simulink model "Q1"  (R2016b)
settings: Solver=VariableStepAuto  StartTime=0.0  StopTime=totaltime  RelTol=1e-3
undefined symbols (not defined in the file): b, st
libraries: xbsIndex_r4 x131
settings Model: Creator=rm101  LastModifiedBy=rm101

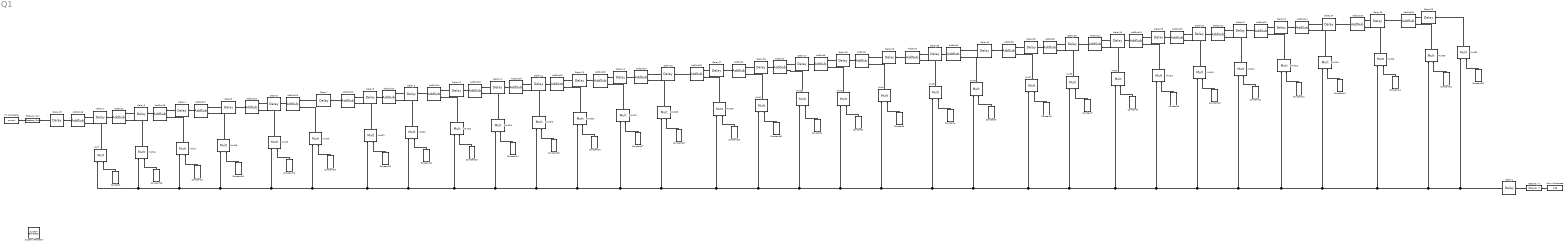
== system Q1 ==
  " System Generator" : xbsIndex_r4/ System Generator  Tag=genX  xilinxfamily=zynq  part=xc7z020  speed=-1  package=clg484  synthesis_tool=Vivado  clock_wrapper=Clock Enables  directory=E:/yg/lab1/generator/Q1_new2  proj_type=Vivado  Synth_file=Vivado Synthesis Defaults  Impl_file=Vivado Implementation Defaults  testbench=off  simulink_period=st  sysclk_period=st*10e6  dcm_input_clock_period=10  incr_netlist=off  trim_vbits=Everywhere in SubSystem  dbl_ovrd=According to Block Masks  core_generation=According to Block Masks  run_coregen=off  deprecated_control=off  eval_field=0  block_type=sysgen
  AddSub{1..31} (31 alike) : xbsIndex_r4/AddSub  mode=Addition  use_carryin=off  use_carryout=off  en=off  latency=0  precision=Full  arith_type=Unsigned  n_bits=16  bin_pt=14  quantization=Truncate  overflow=Wrap  use_behavioral_HDL=off  hw_selection=Fabric  pipelined=off  dbl_ovrd=off  block_type=addsub
  Constant : xbsIndex_r4/Constant  const=b(1)  gui_display_data_type=Fixed-point  arith_type=Signed (2's comp)  n_bits=W  bin_pt=D  preci_type=Single  exp_width=8  frac_width=24  explicit_period=off  period=1  equ=P=C  opselect=C  inp2=PCIN>>17  opr=+  inp1=P  carry=CIN  dbl_ovrd=off  block_type=constant
  Constant1 : xbsIndex_r4/Constant  const=b(17)  gui_display_data_type=Fixed-point  arith_type=Signed (2's comp)  n_bits=W  bin_pt=D  preci_type=Single  exp_width=8  frac_width=24  explicit_period=off  period=1  equ=P=C  opselect=C  inp2=PCIN>>17  opr=+  inp1=P  carry=CIN  dbl_ovrd=off  block_type=constant
  Constant10 : xbsIndex_r4/Constant  const=b(26)  gui_display_data_type=Fixed-point  arith_type=Signed (2's comp)  n_bits=W  bin_pt=D  preci_type=Single  exp_width=8  frac_width=24  explicit_period=off  period=1  equ=P=C  opselect=C  inp2=PCIN>>17  opr=+  inp1=P  carry=CIN  dbl_ovrd=off  block_type=constant
  Constant11 : xbsIndex_r4/Constant  const=b(27)  gui_display_data_type=Fixed-point  arith_type=Signed (2's comp)  n_bits=W  bin_pt=D  preci_type=Single  exp_width=8  frac_width=24  explicit_period=off  period=1  equ=P=C  opselect=C  inp2=PCIN>>17  opr=+  inp1=P  carry=CIN  dbl_ovrd=off  block_type=constant
  Constant12 : xbsIndex_r4/Constant  const=b(28)  gui_display_data_type=Fixed-point  arith_type=Signed (2's comp)  n_bits=W  bin_pt=D  preci_type=Single  exp_width=8  frac_width=24  explicit_period=off  period=1  equ=P=C  opselect=C  inp2=PCIN>>17  opr=+  inp1=P  carry=CIN  dbl_ovrd=off  block_type=constant
  Constant13 : xbsIndex_r4/Constant  const=b(29)  gui_display_data_type=Fixed-point  arith_type=Signed (2's comp)  n_bits=W  bin_pt=D  preci_type=Single  exp_width=8  frac_width=24  explicit_period=off  period=1  equ=P=C  opselect=C  inp2=PCIN>>17  opr=+  inp1=P  carry=CIN  dbl_ovrd=off  block_type=constant
  Constant14 : xbsIndex_r4/Constant  const=b(30)  gui_display_data_type=Fixed-point  arith_type=Signed (2's comp)  n_bits=W  bin_pt=D  preci_type=Single  exp_width=8  frac_width=24  explicit_period=off  period=1  equ=P=C  opselect=C  inp2=PCIN>>17  opr=+  inp1=P  carry=CIN  dbl_ovrd=off  block_type=constant
  Constant16 : xbsIndex_r4/Constant  const=b(2)  gui_display_data_type=Fixed-point  arith_type=Signed (2's comp)  n_bits=W  bin_pt=D  preci_type=Single  exp_width=8  frac_width=24  explicit_period=off  period=1  equ=P=C  opselect=C  inp2=PCIN>>17  opr=+  inp1=P  carry=CIN  dbl_ovrd=off  block_type=constant
  Constant17 : xbsIndex_r4/Constant  const=b(3)  gui_display_data_type=Fixed-point  arith_type=Signed (2's comp)  n_bits=W  bin_pt=D  preci_type=Single  exp_width=8  frac_width=24  explicit_period=off  period=1  equ=P=C  opselect=C  inp2=PCIN>>17  opr=+  inp1=P  carry=CIN  dbl_ovrd=off  block_type=constant
  Constant18 : xbsIndex_r4/Constant  const=b(4)  gui_display_data_type=Fixed-point  arith_type=Signed (2's comp)  n_bits=W  bin_pt=D  preci_type=Single  exp_width=8  frac_width=24  explicit_period=off  period=1  equ=P=C  opselect=C  inp2=PCIN>>17  opr=+  inp1=P  carry=CIN  dbl_ovrd=off  block_type=constant
  Constant19 : xbsIndex_r4/Constant  const=b(5)  gui_display_data_type=Fixed-point  arith_type=Signed (2's comp)  n_bits=W  bin_pt=D  preci_type=Single  exp_width=8  frac_width=24  explicit_period=off  period=1  equ=P=C  opselect=C  inp2=PCIN>>17  opr=+  inp1=P  carry=CIN  dbl_ovrd=off  block_type=constant
  Constant2 : xbsIndex_r4/Constant  const=b(18)  gui_display_data_type=Fixed-point  arith_type=Signed (2's comp)  n_bits=W  bin_pt=D  preci_type=Single  exp_width=8  frac_width=24  explicit_period=off  period=1  equ=P=C  opselect=C  inp2=PCIN>>17  opr=+  inp1=P  carry=CIN  dbl_ovrd=off  block_type=constant
  Constant20 : xbsIndex_r4/Constant  const=b(6)  gui_display_data_type=Fixed-point  arith_type=Signed (2's comp)  n_bits=W  bin_pt=D  preci_type=Single  exp_width=8  frac_width=24  explicit_period=off  period=1  equ=P=C  opselect=C  inp2=PCIN>>17  opr=+  inp1=P  carry=CIN  dbl_ovrd=off  block_type=constant
  Constant21 : xbsIndex_r4/Constant  const=b(7)  gui_display_data_type=Fixed-point  arith_type=Signed (2's comp)  n_bits=W  bin_pt=D  preci_type=Single  exp_width=8  frac_width=24  explicit_period=off  period=1  equ=P=C  opselect=C  inp2=PCIN>>17  opr=+  inp1=P  carry=CIN  dbl_ovrd=off  block_type=constant
  Constant22 : xbsIndex_r4/Constant  const=b(8)  gui_display_data_type=Fixed-point  arith_type=Signed (2's comp)  n_bits=W  bin_pt=D  preci_type=Single  exp_width=8  frac_width=24  explicit_period=off  period=1  equ=P=C  opselect=C  inp2=PCIN>>17  opr=+  inp1=P  carry=CIN  dbl_ovrd=off  block_type=constant
  Constant23 : xbsIndex_r4/Constant  const=b(9)  gui_display_data_type=Fixed-point  arith_type=Signed (2's comp)  n_bits=W  bin_pt=D  preci_type=Single  exp_width=8  frac_width=24  explicit_period=off  period=1  equ=P=C  opselect=C  inp2=PCIN>>17  opr=+  inp1=P  carry=CIN  dbl_ovrd=off  block_type=constant
  Constant24 : xbsIndex_r4/Constant  const=b(10)  gui_display_data_type=Fixed-point  arith_type=Signed (2's comp)  n_bits=W  bin_pt=D  preci_type=Single  exp_width=8  frac_width=24  explicit_period=off  period=1  equ=P=C  opselect=C  inp2=PCIN>>17  opr=+  inp1=P  carry=CIN  dbl_ovrd=off  block_type=constant
  Constant25 : xbsIndex_r4/Constant  const=b(11)  gui_display_data_type=Fixed-point  arith_type=Signed (2's comp)  n_bits=W  bin_pt=D  preci_type=Single  exp_width=8  frac_width=24  explicit_period=off  period=1  equ=P=C  opselect=C  inp2=PCIN>>17  opr=+  inp1=P  carry=CIN  dbl_ovrd=off  block_type=constant
  Constant26 : xbsIndex_r4/Constant  const=b(12)  gui_display_data_type=Fixed-point  arith_type=Signed (2's comp)  n_bits=W  bin_pt=D  preci_type=Single  exp_width=8  frac_width=24  explicit_period=off  period=1  equ=P=C  opselect=C  inp2=PCIN>>17  opr=+  inp1=P  carry=CIN  dbl_ovrd=off  block_type=constant
  Constant27 : xbsIndex_r4/Constant  const=b(13)  gui_display_data_type=Fixed-point  arith_type=Signed (2's comp)  n_bits=W  bin_pt=D  preci_type=Single  exp_width=8  frac_width=24  explicit_period=off  period=1  equ=P=C  opselect=C  inp2=PCIN>>17  opr=+  inp1=P  carry=CIN  dbl_ovrd=off  block_type=constant
  Constant28 : xbsIndex_r4/Constant  const=b(14)  gui_display_data_type=Fixed-point  arith_type=Signed (2's comp)  n_bits=W  bin_pt=D  preci_type=Single  exp_width=8  frac_width=24  explicit_period=off  period=1  equ=P=C  opselect=C  inp2=PCIN>>17  opr=+  inp1=P  carry=CIN  dbl_ovrd=off  block_type=constant
  Constant29 : xbsIndex_r4/Constant  const=b(15)  gui_display_data_type=Fixed-point  arith_type=Signed (2's comp)  n_bits=W  bin_pt=D  preci_type=Single  exp_width=8  frac_width=24  explicit_period=off  period=1  equ=P=C  opselect=C  inp2=PCIN>>17  opr=+  inp1=P  carry=CIN  dbl_ovrd=off  block_type=constant
  Constant3 : xbsIndex_r4/Constant  const=b(19)  gui_display_data_type=Fixed-point  arith_type=Signed (2's comp)  n_bits=W  bin_pt=D  preci_type=Single  exp_width=8  frac_width=24  explicit_period=off  period=1  equ=P=C  opselect=C  inp2=PCIN>>17  opr=+  inp1=P  carry=CIN  dbl_ovrd=off  block_type=constant
  Constant30 : xbsIndex_r4/Constant  const=b(16)  gui_display_data_type=Fixed-point  arith_type=Signed (2's comp)  n_bits=W  bin_pt=D  preci_type=Single  exp_width=8  frac_width=24  explicit_period=off  period=1  equ=P=C  opselect=C  inp2=PCIN>>17  opr=+  inp1=P  carry=CIN  dbl_ovrd=off  block_type=constant
  Constant31 : xbsIndex_r4/Constant  const=b(31)  gui_display_data_type=Fixed-point  arith_type=Signed (2's comp)  n_bits=W  bin_pt=D  preci_type=Single  exp_width=8  frac_width=24  explicit_period=off  period=1  equ=P=C  opselect=C  inp2=PCIN>>17  opr=+  inp1=P  carry=CIN  dbl_ovrd=off  block_type=constant
  Constant32 : xbsIndex_r4/Constant  const=b(32)  gui_display_data_type=Fixed-point  arith_type=Signed (2's comp)  n_bits=W  bin_pt=D  preci_type=Single  exp_width=8  frac_width=24  explicit_period=off  period=1  equ=P=C  opselect=C  inp2=PCIN>>17  opr=+  inp1=P  carry=CIN  dbl_ovrd=off  block_type=constant
  Constant4 : xbsIndex_r4/Constant  const=b(20)  gui_display_data_type=Fixed-point  arith_type=Signed (2's comp)  n_bits=W  bin_pt=D  preci_type=Single  exp_width=8  frac_width=24  explicit_period=off  period=1  equ=P=C  opselect=C  inp2=PCIN>>17  opr=+  inp1=P  carry=CIN  dbl_ovrd=off  block_type=constant
  Constant5 : xbsIndex_r4/Constant  const=b(21)  gui_display_data_type=Fixed-point  arith_type=Signed (2's comp)  n_bits=W  bin_pt=D  preci_type=Single  exp_width=8  frac_width=24  explicit_period=off  period=1  equ=P=C  opselect=C  inp2=PCIN>>17  opr=+  inp1=P  carry=CIN  dbl_ovrd=off  block_type=constant
  Constant6 : xbsIndex_r4/Constant  const=b(22)  gui_display_data_type=Fixed-point  arith_type=Signed (2's comp)  n_bits=W  bin_pt=D  preci_type=Single  exp_width=8  frac_width=24  explicit_period=off  period=1  equ=P=C  opselect=C  inp2=PCIN>>17  opr=+  inp1=P  carry=CIN  dbl_ovrd=off  block_type=constant
  Constant7 : xbsIndex_r4/Constant  const=b(23)  gui_display_data_type=Fixed-point  arith_type=Signed (2's comp)  n_bits=W  bin_pt=D  preci_type=Single  exp_width=8  frac_width=24  explicit_period=off  period=1  equ=P=C  opselect=C  inp2=PCIN>>17  opr=+  inp1=P  carry=CIN  dbl_ovrd=off  block_type=constant
  Constant8 : xbsIndex_r4/Constant  const=b(24)  gui_display_data_type=Fixed-point  arith_type=Signed (2's comp)  n_bits=W  bin_pt=D  preci_type=Single  exp_width=8  frac_width=24  explicit_period=off  period=1  equ=P=C  opselect=C  inp2=PCIN>>17  opr=+  inp1=P  carry=CIN  dbl_ovrd=off  block_type=constant
  Constant9 : xbsIndex_r4/Constant  const=b(25)  gui_display_data_type=Fixed-point  arith_type=Signed (2's comp)  n_bits=W  bin_pt=D  preci_type=Single  exp_width=8  frac_width=24  explicit_period=off  period=1  equ=P=C  opselect=C  inp2=PCIN>>17  opr=+  inp1=P  carry=CIN  dbl_ovrd=off  block_type=constant
  Delay{1..33} (33 alike) : xbsIndex_r4/Delay  rst=off  infoeditControl=Selection of Reset will increase slice count due to use of real FFs and instead of SRLs  en=off  latency=1  reg_retiming=off  dbl_ovrd=off  block_type=delay
  From Workspace : FromWorkspace  VariableName=sig3  SampleTime=0  Interpolate=off  OutputAfterFinalValue=Holding final value
  Gateway In : xbsIndex_r4/Gateway In  gui_display_data_type=Fixed-point  arith_type="Signed  (2's comp)"  n_bits=W  bin_pt=D  preci_type=Single  exp_width=8  frac_width=24  rows=1  columns=1  quantization="Round  (unbiased: +/- Inf)"  overflow=Flag as error  period=st  UseAsADC=off  ADCChannel='1'  interface=None  automatic_assignment=on  address_offset=hex2dec('00')  intf_name=''  intf_description=''  default_value=0  timing_constraint=None  locs_specified=off  LOCs={}  io_standard={}  inherit_from_input=off  hdl_port=on  dbl_ovrd=off  block_type=gatewayin
  Gateway Out : xbsIndex_r4/Gateway Out  inherit_from_input=off  hdl_port=on  rows=1  columns=1  UseAsDAC=off  DACChannel='1'  interface=None  automatic_assignment=on  address_offset=hex2dec('00')  intf_name=''  intf_description=''  timing_constraint=None  locs_specified=off  LOCs={}  io_standard={}  block_type=gatewayout
  Mult{,1..30,32} (32 alike) : xbsIndex_r4/Mult  precision=User Defined  arith_type="Signed  (2's comp)"  n_bits=W  bin_pt=D  quantization="Round  (unbiased: +/- Inf)"  overflow=Flag as error  en=off  latency=0  use_behavioral_HDL=off  opt=Speed  use_embedded=on  optimum_pipeline=off  pipeline=on  dbl_ovrd=off  use_rpm=on  placement_style=Triangular  block_type=mult
  To Workspace : ToWorkspace  VariableName=simout  SaveFormat=Timeseries  SampleTime=-1
  wires:
  Constant/1 -> Mult/2
  Gateway Out/1 -> To Workspace/1
  From Workspace/1 -> Gateway In/1
  Delay15/1 -> Gateway Out/1
  AddSub16/1 -> Delay15/1
  Mult/1 -> AddSub16/2
  Constant16/1 -> Mult16/2
  Mult16/1 -> AddSub1/2
  AddSub1/1 -> Delay2/1
  Constant17/1 -> Mult17/2
  Mult17/1 -> AddSub18/2
  Constant18/1 -> Mult18/2
  Mult18/1 -> AddSub17/2
  AddSub17/1 -> Delay4/1
  AddSub18/1 -> Delay3/1
  Constant19/1 -> Mult19/2
  Mult19/1 -> AddSub20/2
  Constant20/1 -> Mult20/2
  Mult20/1 -> AddSub19/2
  AddSub19/1 -> Delay6/1
  AddSub20/1 -> Delay5/1
  Constant21/1 -> Mult21/2
  Mult21/1 -> AddSub22/2
  Constant22/1 -> Mult22/2
  Mult22/1 -> AddSub21/2
  AddSub21/1 -> Delay8/1
  AddSub22/1 -> Delay7/1
  Constant23/1 -> Mult23/2
  Mult23/1 -> AddSub24/2
  Constant24/1 -> Mult24/2
  Mult24/1 -> AddSub23/2
  AddSub23/1 -> Delay10/1
  Constant25/1 -> Mult25/2
  Mult25/1 -> AddSub26/2
  Constant26/1 -> Mult26/2
  Mult26/1 -> AddSub25/2
  AddSub25/1 -> Delay12/1
  AddSub26/1 -> Delay11/1
  Constant27/1 -> Mult27/2
  Mult27/1 -> AddSub28/2
  Constant28/1 -> Mult28/2
  Mult28/1 -> AddSub27/2
  AddSub27/1 -> Delay14/1
  AddSub28/1 -> Delay13/1
  Constant29/1 -> Mult29/2
  Mult29/1 -> AddSub30/2
  AddSub30/1 -> Delay16/1
  AddSub24/1 -> Delay9/1
  Gateway In/1 -> Delay1/1
  Delay2/1 -> AddSub16/1
  Delay3/1 -> AddSub1/1
  Delay4/1 -> AddSub18/1
  Delay5/1 -> AddSub17/1
  Delay6/1 -> AddSub20/1
  Delay7/1 -> AddSub19/1
  Delay8/1 -> AddSub22/1
  Delay9/1 -> AddSub21/1
  Delay10/1 -> AddSub24/1
  Delay11/1 -> AddSub23/1
  Delay12/1 -> AddSub26/1
  Delay13/1 -> AddSub25/1
  Delay14/1 -> AddSub28/1
  Delay16/1 -> AddSub27/1
  Delay17/1 -> AddSub30/1
  Constant30/1 -> Mult1/2
  ? -> ?
  AddSub3/1 -> Delay17/1
  Mult1/1 -> AddSub3/2
  Constant1/1 -> Mult2/2
  Mult2/1 -> AddSub2/2
  AddSub2/1 -> Delay26/1
  Constant2/1 -> Mult3/2
  Mult3/1 -> AddSub5/2
  Constant3/1 -> Mult4/2
  Mult4/1 -> AddSub4/2
  AddSub4/1 -> Delay28/1
  AddSub5/1 -> Delay27/1
  Constant4/1 -> Mult5/2
  Mult5/1 -> AddSub7/2
  Constant5/1 -> Mult6/2
  Mult6/1 -> AddSub6/2
  AddSub6/1 -> Delay30/1
  AddSub7/1 -> Delay29/1
  Constant6/1 -> Mult7/2
  Mult7/1 -> AddSub9/2
  Constant7/1 -> Mult8/2
  Mult8/1 -> AddSub8/2
  AddSub8/1 -> Delay32/1
  AddSub9/1 -> Delay31/1
  Constant8/1 -> Mult9/2
  Mult9/1 -> AddSub11/2
  Constant9/1 -> Mult10/2
  Mult10/1 -> AddSub10/2
  AddSub10/1 -> Delay18/1
  Constant10/1 -> Mult11/2
  Mult11/1 -> AddSub13/2
  Constant11/1 -> Mult12/2
  Mult12/1 -> AddSub12/2
  AddSub12/1 -> Delay20/1
  AddSub13/1 -> Delay19/1
  Constant12/1 -> Mult13/2
  Mult13/1 -> AddSub15/2
  Constant13/1 -> Mult14/2
  Mult14/1 -> AddSub14/2
  AddSub14/1 -> Delay22/1
  AddSub15/1 -> Delay21/1
  Constant14/1 -> Mult15/2
  Mult15/1 -> AddSub29/2
  AddSub29/1 -> Delay24/1
  AddSub11/1 -> Delay33/1
  Delay26/1 -> AddSub3/1
  Delay27/1 -> AddSub2/1
  Delay28/1 -> AddSub5/1
  Delay29/1 -> AddSub4/1
  Delay30/1 -> AddSub7/1
  Delay31/1 -> AddSub6/1
  Delay32/1 -> AddSub9/1
  Delay33/1 -> AddSub8/1
  Delay18/1 -> AddSub11/1
  Delay19/1 -> AddSub10/1
  Delay20/1 -> AddSub13/1
  Delay21/1 -> AddSub12/1
  Delay22/1 -> AddSub15/1
  Delay24/1 -> AddSub14/1
  Delay25/1 -> AddSub29/1
  Constant31/1 -> Mult30/2
  Mult30/1 -> AddSub31/2
  Constant32/1 -> Mult32/2
  Mult32/1 -> Delay23/1
  Delay23/1 -> AddSub31/1
  Delay1/1 -> Mult32/1, Mult30/1, Mult15/1, Mult14/1, Mult13/1, Mult12/1, Mult11/1, Mult10/1, Mult9/1, Mult8/1, Mult7/1, Mult6/1, Mult5/1, Mult4/1, Mult3/1, Mult2/1, Mult1/1, Mult29/1, Mult28/1, Mult27/1, Mult26/1, Mult25/1, Mult24/1, Mult23/1, Mult22/1, Mult21/1, Mult20/1, Mult19/1, Mult18/1, Mult17/1, Mult16/1, Mult/1
  AddSub31/1 -> Delay25/1
